simulink model "fulldeminsionscope"  (R2016b)
settings: Solver=VariableStepAuto  StartTime=0.0  StopTime=20.0  RelTol=1e-3
settings Model: Creator=gz199  LastModifiedBy=gz199

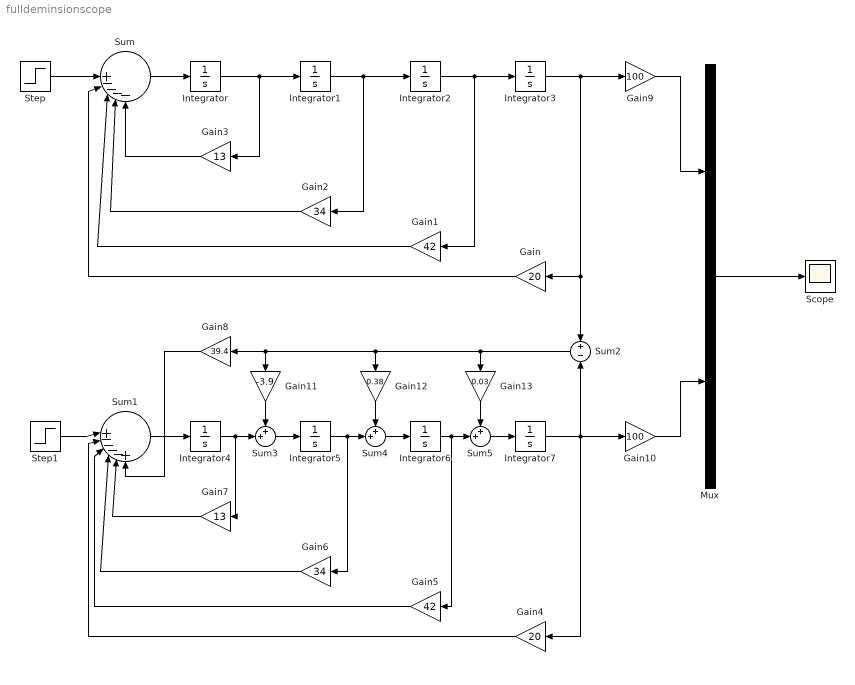
== system fulldeminsionscope ==
  Gain : Gain  Gain=20
  Gain1 : Gain  Gain=42
  Gain10 : Gain  Gain=100
  Gain11 : Gain  Gain=-3.9
  Gain12 : Gain  Gain=0.38
  Gain13 : Gain  Gain=0.03
  Gain2 : Gain  Gain=34
  Gain3 : Gain  Gain=13
  Gain4 : Gain  Gain=20
  Gain5 : Gain  Gain=42
  Gain6 : Gain  Gain=34
  Gain7 : Gain  Gain=13
  Gain8 : Gain  Gain=39.4
  Gain9 : Gain  Gain=100
  Integrator{,1..7} (8 alike) : Integrator
  Mux : Mux  Inputs=2
  Scope : Scope
  Step : Step  Time=0  SampleTime=0
  Step1 : Step  Time=8  SampleTime=0
  Sum : Sum  Inputs=||||+----
  Sum1 : Sum  Inputs=||||+----+
  Sum2 : Sum  Inputs=+-
  Sum3 : Sum  Inputs=++|
  Sum4 : Sum  Inputs=++|
  Sum5 : Sum  Inputs=++|
  wires:
  Integrator/1 -> Gain3/1, Integrator1/1
  Integrator1/1 -> Gain2/1, Integrator2/1
  Integrator2/1 -> Gain1/1, Integrator3/1
  Sum/1 -> Integrator/1
  Gain/1 -> Sum/2
  Gain3/1 -> Sum/5
  Gain2/1 -> Sum/4
  Gain1/1 -> Sum/3
  Integrator3/1 -> Sum2/1, Gain/1, Gain9/1
  Step/1 -> Sum/1
  Sum1/1 -> Integrator4/1
  Gain4/1 -> Sum1/2
  Gain7/1 -> Sum1/5
  Gain6/1 -> Sum1/4
  Gain5/1 -> Sum1/3
  Integrator7/1 -> Gain10/1, Gain4/1, Sum2/2
  Step1/1 -> Sum1/1
  Sum2/1 -> Gain12/1, Gain11/1, Gain8/1, Gain13/1
  Gain8/1 -> Sum1/6
  Gain9/1 -> Mux/1
  Gain10/1 -> Mux/2
  Sum3/1 -> Integrator5/1
  Integrator4/1 -> Gain7/1, Sum3/2
  Sum4/1 -> Integrator6/1
  Sum5/1 -> Integrator7/1
  Integrator6/1 -> Gain5/1, Sum5/2
  Integrator5/1 -> Gain6/1, Sum4/2
  Gain11/1 -> Sum3/1
  Gain12/1 -> Sum4/1
  Gain13/1 -> Sum5/1
  Mux/1 -> Scope/1
